simulink model "ball"  (Simulink 8.9)
settings: Solver=ode45  StartTime=0.0  StopTime=10.0  RelTol=1e-2  EnableMultiTasking=on
settings Model: Creator=Knut  LastModifiedBy=Knut  ExtModeTrigMode=oneshot  ExtModeArmWhenConnect=off
settings SolverCC: ZeroCrossControl=DisableAll
settings DataIOCC: LimitDataPoints=off
settings OptimizationCC: BlockReduction=off  BooleanDataType=off  LifeSpan=auto
settings DebuggingCC: SaveWithParameterizedLinksMsg=none  SignalResolutionControl=TryResolveAllWithWarning  MultiTaskDSMMsg=warning  MultiTaskCondExecSysMsg=none  FcnCallInpInsideContextMsg=error  StateNameClashWarn=none  StrictBusMsg=None  SFUnexpectedBacktrackingDiag=error  SFNoUnconditionalDefaultTransitionDiag=error  SFExecutionAtInitializationDiag=warning
settings HardwareCC: ProdBitPerPointer=64  ProdBitPerSizeT=64  ProdBitPerPtrDiffT=64  ProdLargestAtomicFloat=Float  ProdIntDivRoundTo=Zero  ProdEndianess=LittleEndian  ProdWordSize=64  ProdHWDeviceType=Intel->x86-64 (Windows64)  TargetUnknown=on
settings GRTTargetCC: GeneratePreprocessorConditionals=Use local settings
settings ConfigComp: CovMetricSettings=dwe

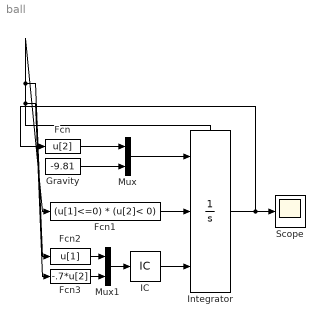
== system ball ==
  Fcn : Fcn  Expr=u[2]
  Fcn1 : Fcn  Expr=(u[1]<=0) * (u[2]< 0)
  Fcn2 : Fcn  Expr=u[1]
  Fcn3 : Fcn  Expr=-.7*u[2]
  Gravity : Constant  Value=-9.81
  IC : InitialCondition  Value=[10;5]
  Integrator : Integrator  ExternalReset=rising  InitialConditionSource=external  LimitOutput=on  LowerSaturationLimit=[0;-inf]  ShowStatePort=on
  Mux : Mux  Inputs=2
  Mux1 : Mux  Inputs=2
  Scope : Scope
  wires:
  Fcn1/1 -> Integrator/2
  Mux/1 -> Integrator/1
  Gravity/1 -> Mux/2
  Fcn/1 -> Mux/1
  Fcn3/1 -> Mux1/2
  Fcn2/1 -> Mux1/1
  Integrator/State -> Fcn3/1, Fcn2/1, Fcn1/1
  Mux1/1 -> IC/1
  IC/1 -> Integrator/3
  Integrator/1 -> Scope/1, Fcn/1
